simulink model "pmsm_electrical_id_waveform_model"  (R2023b)
settings: Solver=FixedStepDiscrete  StartTime=0.0  StopTime=0.45  FixedStep=5e-5  RelTol=1e-3
model workspace (MAT data in the model file):
  angle_delta = [0 0.0001 0.0002 0.0003 0.0004 0.0005 0.0006 0.0007 0.0008 0.0009 0.001 0.0011 ... (8000 elements, 4000x2)]
  angle_encoder = [0 0.0001 0.0002 0.0003 0.0004 0.0005 0.0006 0.0007 0.0008 0.0009 0.001 0.0011 ... (8000 elements, 4000x2)]
  angle_residual = [0 0.0001 0.0002 0.0003 0.0004 0.0005 0.0006 0.0007 0.0008 0.0009 0.001 0.0011 ... (8000 elements, 4000x2)]
  angle_sensorless = [0 0.0001 0.0002 0.0003 0.0004 0.0005 0.0006 0.0007 0.0008 0.0009 0.001 0.0011 ... (8000 elements, 4000x2)]
  angle_true = [0 0.0001 0.0002 0.0003 0.0004 0.0005 0.0006 0.0007 0.0008 0.0009 0.001 0.0011 ... (8000 elements, 4000x2)]
  flux_id = [0 0.001 0.002 0.003 0.004 0.005 0.006 0.007 0.008 0.009 0.01 0.011 ... (2000 elements, 1000x2)]
  flux_iq = [0 0.001 0.002 0.003 0.004 0.005 0.006 0.007 0.008 0.009 0.01 0.011 ... (2000 elements, 1000x2)]
  flux_psi_est = [0 0.001 0.002 0.003 0.004 0.005 0.006 0.007 0.008 0.009 0.01 0.011 ... (2000 elements, 1000x2)]
  flux_vq = [0 0.001 0.002 0.003 0.004 0.005 0.006 0.007 0.008 0.009 0.01 0.011 ... (2000 elements, 1000x2)]
  flux_we = [0 0.001 0.002 0.003 0.004 0.005 0.006 0.007 0.008 0.009 0.01 0.011 ... (2000 elements, 1000x2)]
  step_d_current = [0 5e-05 0.0001 0.00015 0.0002 0.00025 0.0003 0.00035 0.0004 0.00045 0.0005 0.00055 ... (2002 elements, 1001x2)]
  step_d_voltage = [0 5e-05 0.0001 0.00015 0.0002 0.00025 0.0003 0.00035 0.0004 0.00045 0.0005 0.00055 ... (2002 elements, 1001x2)]
  step_q_current = [0 5e-05 0.0001 0.00015 0.0002 0.00025 0.0003 0.00035 0.0004 0.00045 0.0005 0.00055 ... (2002 elements, 1001x2)]
  step_q_voltage = [0 5e-05 0.0001 0.00015 0.0002 0.00025 0.0003 0.00035 0.0004 0.00045 0.0005 0.00055 ... (2002 elements, 1001x2)]
(part 2 of 2)

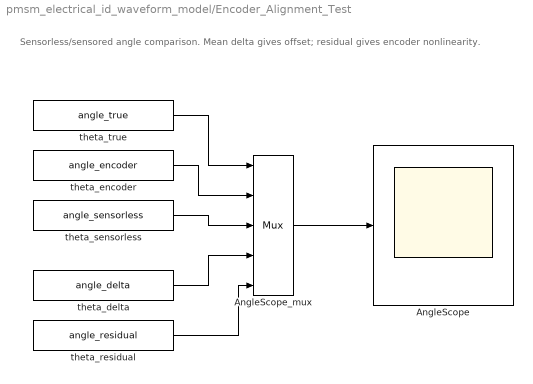
== system pmsm_electrical_id_waveform_model/Encoder_Alignment_Test ==
  note: Sensorless/sensored angle comparison. Mean delta gives offset; residual gives encoder nonlinearity.
  AngleScope : Scope
  AngleScope_mux : Mux  Inputs=5
  theta_delta : FromWorkspace  VariableName=angle_delta
  theta_encoder : FromWorkspace  VariableName=angle_encoder
  theta_residual : FromWorkspace  VariableName=angle_residual
  theta_sensorless : FromWorkspace  VariableName=angle_sensorless
  theta_true : FromWorkspace  VariableName=angle_true
  wires:
  AngleScope_mux/1 -> AngleScope/1
  theta_true/1 -> AngleScope_mux/1
  theta_encoder/1 -> AngleScope_mux/2
  theta_sensorless/1 -> AngleScope_mux/3
  theta_delta/1 -> AngleScope_mux/4
  theta_residual/1 -> AngleScope_mux/5

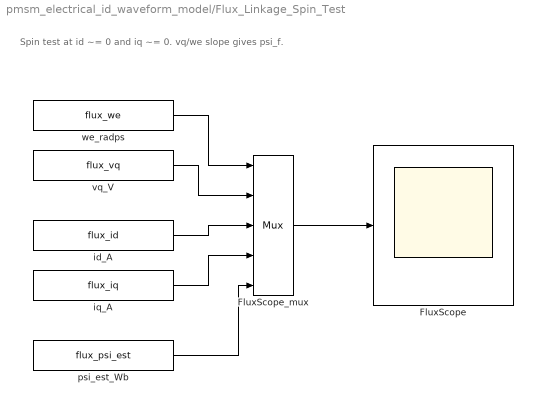
== system pmsm_electrical_id_waveform_model/Flux_Linkage_Spin_Test ==
  note: Spin test at id ~= 0 and iq ~= 0. vq/we slope gives psi_f.
  FluxScope : Scope
  FluxScope_mux : Mux  Inputs=5
  id_A : FromWorkspace  VariableName=flux_id
  iq_A : FromWorkspace  VariableName=flux_iq
  psi_est_Wb : FromWorkspace  VariableName=flux_psi_est
  vq_V : FromWorkspace  VariableName=flux_vq
  we_radps : FromWorkspace  VariableName=flux_we
  wires:
  FluxScope_mux/1 -> FluxScope/1
  we_radps/1 -> FluxScope_mux/1
  vq_V/1 -> FluxScope_mux/2
  id_A/1 -> FluxScope_mux/3
  iq_A/1 -> FluxScope_mux/4
  psi_est_Wb/1 -> FluxScope_mux/5

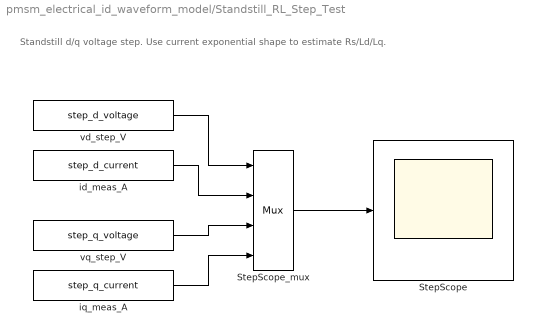
== system pmsm_electrical_id_waveform_model/Standstill_RL_Step_Test ==
  note: Standstill d/q voltage step. Use current exponential shape to estimate Rs/Ld/Lq.
  StepScope : Scope
  StepScope_mux : Mux
  id_meas_A : FromWorkspace  VariableName=step_d_current
  iq_meas_A : FromWorkspace  VariableName=step_q_current
  vd_step_V : FromWorkspace  VariableName=step_d_voltage
  vq_step_V : FromWorkspace  VariableName=step_q_voltage
  wires:
  StepScope_mux/1 -> StepScope/1
  vd_step_V/1 -> StepScope_mux/1
  id_meas_A/1 -> StepScope_mux/2
  vq_step_V/1 -> StepScope_mux/3
  iq_meas_A/1 -> StepScope_mux/4
